simulink model "FaceDet_x4"  (Simulink 7.7)
settings: Solver=FixedStepDiscrete  StartTime=0  StopTime=10  RelTol=1e-3
libraries: simulink x257
(part 2 of 5)

== system FaceDet_x4/FaceDetection/FU/MemBank ==
  LineIdxsLatch : Inport
  LineIdxsExt : Inport  Port=2
  NodeWeightsCtrlRdAdr : Inport  Port=3
  NodeWeightsCtrlWrAdr : Inport  Port=4
  NodeWeightsCtrlEn : Inport  Port=5
  NodeWeightsExt : Inport  Port=6
  FeatureDataLatch : Inport  Port=7
  FeatureDataExt : Inport  Port=8
  WeakTreshLatch : Inport  Port=9
  WeakTreshExt : Inport  Port=10
  StrongTreshLatch : Inport  Port=11
  StrongTreshExt : Inport  Port=12
  FeatureDataMem : Subsystem
  LineIdxsMem : Subsystem
  NodeWeightsMem : Subsystem
  StrongTreshReg : simulink/Additional Math & Discrete/Additional Discrete/Unit Delay Enabled  SystemSampleTime=-1  vinit=0  tsamp=-1
  WeakTreshMem : Subsystem
  LineIdxs : Outport
  NodeWeights : Outport  Port=2
  FeatureData : Outport  Port=3
  StrongTresh : Outport  Port=4
  WeakTresh : Outport  Port=5
  wires:
  LineIdxsLatch/1 -> LineIdxsMem/1(LineIdxsLatch)
  LineIdxsExt/1 -> LineIdxsMem/2(LineIdxsExt)
  LineIdxsMem/1(LineIdxs) -> LineIdxs/1
  NodeWeightsCtrlRdAdr/1 -> NodeWeightsMem/1(NodeWeightsCtrlRdAdr)
  NodeWeightsExt/1 -> NodeWeightsMem/4(NodeWeightsExt)
  NodeWeightsMem/1(NodeWeights) -> NodeWeights/1
  FeatureDataMem/1(FeatureData) -> FeatureData/1
  FeatureDataLatch/1 -> FeatureDataMem/1(FeatureDataLatch)
  FeatureDataExt/1 -> FeatureDataMem/2(FeatureDataExt)
  WeakTreshMem/1(WeakTresh) -> WeakTresh/1
  WeakTreshLatch/1 -> WeakTreshMem/1(WeakTreshLatch)
  WeakTreshExt/1 -> WeakTreshMem/2(WeakTreshExt)
  StrongTreshReg/1 -> StrongTresh/1
  NodeWeightsCtrlEn/1 -> NodeWeightsMem/3(NodeWeightsCtrlEn)
  StrongTreshLatch/1 -> StrongTreshReg/2
  StrongTreshExt/1 -> StrongTreshReg/1
  NodeWeightsCtrlWrAdr/1 -> NodeWeightsMem/2(NodeWeightsCtrlWrAdr)

== system FaceDet_x4/FaceDetection/DU/SplittedDL1/DelLine0_SPRAM_512x5 ==
  addr : Inport
  din : Inport  Port=2
  we : Inport  Port=3  OutDataTypeStr=boolean
  AddressSpec : SignalSpecification  OutDataTypeStr=fixdt(0,depth_bits,0)  Dimensions=1
  And : Logic  AllPortsSameDT=off  OutDataTypeStr=boolean
  DataSpec : SignalSpecification  OutDataTypeStr=fixdt(0,width_bits,0)  Dimensions=1
  Switch1 : Switch  Criteria=u2 ~= 0
  convert : DataTypeConversion  OutDataTypeStr=uint16
  din_d : UnitDelay  SampleTime=-1
  dout_type : Constant  Value=dout_type
  is_new : simulink/Logic and Bit Operations/Compare To Constant  SystemSampleTime=-1  relop===  const=1  LogicOutDataTypeMode=boolean  ZeroCross=off
  ram : UnitDelay  SampleTime=-1
  ram_data : UnitDelay  SampleTime=-1
  select : Selector  IndexMode=Zero-based  InputPortWidth=2^depth_bits  IndexOptions=Index vector (port)  Indices=[1 3]  OutputSizes=1
  switch : Switch  Criteria=u2 ~= 0
  we_d : UnitDelay  SampleTime=-1
  wr_port : Assignment  IndexMode=Zero-based  IndexOptions=Index vector (port)  Indices=1  OutputSizes=[1 1]
  dout : Outport
  wires:
  wr_port/1 -> switch/1
  switch/1 -> ram/1
  ram/1 -> switch/3, wr_port/1, select/1
  din/1 -> DataSpec/1
  we/1 -> switch/2, we_d/1
  addr/1 -> AddressSpec/1
  select/1 -> ram_data/1
  convert/1 -> wr_port/3, select/2
  AddressSpec/1 -> convert/1
  Switch1/1 -> dout/1
  din_d/1 -> Switch1/1
  And/1 -> Switch1/2
  ram_data/1 -> Switch1/3
  dout_type/1 -> is_new/1
  is_new/1 -> And/2
  we_d/1 -> And/1
  DataSpec/1 -> wr_port/2, din_d/1

== system FaceDet_x4/FaceDetection/DU/SplittedDL1/DelLine1_SPRAM_512x5 ==
  addr : Inport
  din : Inport  Port=2
  we : Inport  Port=3  OutDataTypeStr=boolean
  AddressSpec : SignalSpecification  OutDataTypeStr=fixdt(0,depth_bits,0)  Dimensions=1
  And : Logic  AllPortsSameDT=off  OutDataTypeStr=boolean
  DataSpec : SignalSpecification  OutDataTypeStr=fixdt(0,width_bits,0)  Dimensions=1
  Switch1 : Switch  Criteria=u2 ~= 0
  convert : DataTypeConversion  OutDataTypeStr=uint16
  din_d : UnitDelay  SampleTime=-1
  dout_type : Constant  Value=dout_type
  is_new : simulink/Logic and Bit Operations/Compare To Constant  SystemSampleTime=-1  relop===  const=1  LogicOutDataTypeMode=boolean  ZeroCross=off
  ram : UnitDelay  SampleTime=-1
  ram_data : UnitDelay  SampleTime=-1
  select : Selector  IndexMode=Zero-based  InputPortWidth=2^depth_bits  IndexOptions=Index vector (port)  Indices=[1 3]  OutputSizes=1
  switch : Switch  Criteria=u2 ~= 0
  we_d : UnitDelay  SampleTime=-1
  wr_port : Assignment  IndexMode=Zero-based  IndexOptions=Index vector (port)  Indices=1  OutputSizes=[1 1]
  dout : Outport
  wires:
  DataSpec/1 -> din_d/1, wr_port/2
  we_d/1 -> And/1
  is_new/1 -> And/2
  dout_type/1 -> is_new/1
  ram_data/1 -> Switch1/3
  And/1 -> Switch1/2
  din_d/1 -> Switch1/1
  Switch1/1 -> dout/1
  AddressSpec/1 -> convert/1
  convert/1 -> select/2, wr_port/3
  select/1 -> ram_data/1
  addr/1 -> AddressSpec/1
  we/1 -> we_d/1, switch/2
  din/1 -> DataSpec/1
  ram/1 -> select/1, wr_port/1, switch/3
  switch/1 -> ram/1
  wr_port/1 -> switch/1

== system FaceDet_x4/FaceDetection/DU/SplittedDL1/DelLine2_SPRAM_512x5 ==
  addr : Inport
  din : Inport  Port=2
  we : Inport  Port=3  OutDataTypeStr=boolean
  AddressSpec : SignalSpecification  OutDataTypeStr=fixdt(0,depth_bits,0)  Dimensions=1
  And : Logic  AllPortsSameDT=off  OutDataTypeStr=boolean
  DataSpec : SignalSpecification  OutDataTypeStr=fixdt(0,width_bits,0)  Dimensions=1
  Switch1 : Switch  Criteria=u2 ~= 0
  convert : DataTypeConversion  OutDataTypeStr=uint16
  din_d : UnitDelay  SampleTime=-1
  dout_type : Constant  Value=dout_type
  is_new : simulink/Logic and Bit Operations/Compare To Constant  SystemSampleTime=-1  relop===  const=1  LogicOutDataTypeMode=boolean  ZeroCross=off
  ram : UnitDelay  SampleTime=-1
  ram_data : UnitDelay  SampleTime=-1
  select : Selector  IndexMode=Zero-based  InputPortWidth=2^depth_bits  IndexOptions=Index vector (port)  Indices=[1 3]  OutputSizes=1
  switch : Switch  Criteria=u2 ~= 0
  we_d : UnitDelay  SampleTime=-1
  wr_port : Assignment  IndexMode=Zero-based  IndexOptions=Index vector (port)  Indices=1  OutputSizes=[1 1]
  dout : Outport
  wires:
  wr_port/1 -> switch/1
  switch/1 -> ram/1
  ram/1 -> switch/3, wr_port/1, select/1
  din/1 -> DataSpec/1
  we/1 -> switch/2, we_d/1
  addr/1 -> AddressSpec/1
  select/1 -> ram_data/1
  convert/1 -> wr_port/3, select/2
  AddressSpec/1 -> convert/1
  Switch1/1 -> dout/1
  din_d/1 -> Switch1/1
  And/1 -> Switch1/2
  ram_data/1 -> Switch1/3
  dout_type/1 -> is_new/1
  is_new/1 -> And/2
  we_d/1 -> And/1
  DataSpec/1 -> wr_port/2, din_d/1

== system FaceDet_x4/FaceDetection/DU/SplittedDL1/DelLine3_SPRAM_512x5 ==
  addr : Inport
  din : Inport  Port=2
  we : Inport  Port=3  OutDataTypeStr=boolean
  AddressSpec : SignalSpecification  OutDataTypeStr=fixdt(0,depth_bits,0)  Dimensions=1
  And : Logic  AllPortsSameDT=off  OutDataTypeStr=boolean
  DataSpec : SignalSpecification  OutDataTypeStr=fixdt(0,width_bits,0)  Dimensions=1
  Switch1 : Switch  Criteria=u2 ~= 0
  convert : DataTypeConversion  OutDataTypeStr=uint16
  din_d : UnitDelay  SampleTime=-1
  dout_type : Constant  Value=dout_type
  is_new : simulink/Logic and Bit Operations/Compare To Constant  SystemSampleTime=-1  relop===  const=1  LogicOutDataTypeMode=boolean  ZeroCross=off
  ram : UnitDelay  SampleTime=-1
  ram_data : UnitDelay  SampleTime=-1
  select : Selector  IndexMode=Zero-based  InputPortWidth=2^depth_bits  IndexOptions=Index vector (port)  Indices=[1 3]  OutputSizes=1
  switch : Switch  Criteria=u2 ~= 0
  we_d : UnitDelay  SampleTime=-1
  wr_port : Assignment  IndexMode=Zero-based  IndexOptions=Index vector (port)  Indices=1  OutputSizes=[1 1]
  dout : Outport
  wires:
  DataSpec/1 -> din_d/1, wr_port/2
  we_d/1 -> And/1
  is_new/1 -> And/2
  dout_type/1 -> is_new/1
  ram_data/1 -> Switch1/3
  And/1 -> Switch1/2
  din_d/1 -> Switch1/1
  Switch1/1 -> dout/1
  AddressSpec/1 -> convert/1
  convert/1 -> select/2, wr_port/3
  select/1 -> ram_data/1
  addr/1 -> AddressSpec/1
  we/1 -> we_d/1, switch/2
  din/1 -> DataSpec/1
  ram/1 -> select/1, wr_port/1, switch/3
  switch/1 -> ram/1
  wr_port/1 -> switch/1

== system FaceDet_x4/FaceDetection/DU/SplittedDL1/DelLine4_SPRAM_512x5 ==
  addr : Inport
  din : Inport  Port=2
  we : Inport  Port=3  OutDataTypeStr=boolean
  AddressSpec : SignalSpecification  OutDataTypeStr=fixdt(0,depth_bits,0)  Dimensions=1
  And : Logic  AllPortsSameDT=off  OutDataTypeStr=boolean
  DataSpec : SignalSpecification  OutDataTypeStr=fixdt(0,width_bits,0)  Dimensions=1
  Switch1 : Switch  Criteria=u2 ~= 0
  convert : DataTypeConversion  OutDataTypeStr=uint16
  din_d : UnitDelay  SampleTime=-1
  dout_type : Constant  Value=dout_type
  is_new : simulink/Logic and Bit Operations/Compare To Constant  SystemSampleTime=-1  relop===  const=1  LogicOutDataTypeMode=boolean  ZeroCross=off
  ram : UnitDelay  SampleTime=-1
  ram_data : UnitDelay  SampleTime=-1
  select : Selector  IndexMode=Zero-based  InputPortWidth=2^depth_bits  IndexOptions=Index vector (port)  Indices=[1 3]  OutputSizes=1
  switch : Switch  Criteria=u2 ~= 0
  we_d : UnitDelay  SampleTime=-1
  wr_port : Assignment  IndexMode=Zero-based  IndexOptions=Index vector (port)  Indices=1  OutputSizes=[1 1]
  dout : Outport
  wires:
  wr_port/1 -> switch/1
  switch/1 -> ram/1
  ram/1 -> switch/3, wr_port/1, select/1
  din/1 -> DataSpec/1
  we/1 -> switch/2, we_d/1
  addr/1 -> AddressSpec/1
  select/1 -> ram_data/1
  convert/1 -> wr_port/3, select/2
  AddressSpec/1 -> convert/1
  Switch1/1 -> dout/1
  din_d/1 -> Switch1/1
  And/1 -> Switch1/2
  ram_data/1 -> Switch1/3
  dout_type/1 -> is_new/1
  is_new/1 -> And/2
  we_d/1 -> And/1
  DataSpec/1 -> wr_port/2, din_d/1

== system FaceDet_x4/FaceDetection/DU/SplittedDL1/DelLine5_SPRAM_512x5 ==
  addr : Inport
  din : Inport  Port=2
  we : Inport  Port=3  OutDataTypeStr=boolean
  AddressSpec : SignalSpecification  OutDataTypeStr=fixdt(0,depth_bits,0)  Dimensions=1
  And : Logic  AllPortsSameDT=off  OutDataTypeStr=boolean
  DataSpec : SignalSpecification  OutDataTypeStr=fixdt(0,width_bits,0)  Dimensions=1
  Switch1 : Switch  Criteria=u2 ~= 0
  convert : DataTypeConversion  OutDataTypeStr=uint16
  din_d : UnitDelay  SampleTime=-1
  dout_type : Constant  Value=dout_type
  is_new : simulink/Logic and Bit Operations/Compare To Constant  SystemSampleTime=-1  relop===  const=1  LogicOutDataTypeMode=boolean  ZeroCross=off
  ram : UnitDelay  SampleTime=-1
  ram_data : UnitDelay  SampleTime=-1
  select : Selector  IndexMode=Zero-based  InputPortWidth=2^depth_bits  IndexOptions=Index vector (port)  Indices=[1 3]  OutputSizes=1
  switch : Switch  Criteria=u2 ~= 0
  we_d : UnitDelay  SampleTime=-1
  wr_port : Assignment  IndexMode=Zero-based  IndexOptions=Index vector (port)  Indices=1  OutputSizes=[1 1]
  dout : Outport
  wires:
  DataSpec/1 -> din_d/1, wr_port/2
  we_d/1 -> And/1
  is_new/1 -> And/2
  dout_type/1 -> is_new/1
  ram_data/1 -> Switch1/3
  And/1 -> Switch1/2
  din_d/1 -> Switch1/1
  Switch1/1 -> dout/1
  AddressSpec/1 -> convert/1
  convert/1 -> select/2, wr_port/3
  select/1 -> ram_data/1
  addr/1 -> AddressSpec/1
  we/1 -> we_d/1, switch/2
  din/1 -> DataSpec/1
  ram/1 -> select/1, wr_port/1, switch/3
  switch/1 -> ram/1
  wr_port/1 -> switch/1

== system FaceDet_x4/FaceDetection/DU/SplittedDL1/DelLine6_SPRAM_512x5 ==
  addr : Inport
  din : Inport  Port=2
  we : Inport  Port=3  OutDataTypeStr=boolean
  AddressSpec : SignalSpecification  OutDataTypeStr=fixdt(0,depth_bits,0)  Dimensions=1
  And : Logic  AllPortsSameDT=off  OutDataTypeStr=boolean
  DataSpec : SignalSpecification  OutDataTypeStr=fixdt(0,width_bits,0)  Dimensions=1
  Switch1 : Switch  Criteria=u2 ~= 0
  convert : DataTypeConversion  OutDataTypeStr=uint16
  din_d : UnitDelay  SampleTime=-1
  dout_type : Constant  Value=dout_type
  is_new : simulink/Logic and Bit Operations/Compare To Constant  SystemSampleTime=-1  relop===  const=1  LogicOutDataTypeMode=boolean  ZeroCross=off
  ram : UnitDelay  SampleTime=-1
  ram_data : UnitDelay  SampleTime=-1
  select : Selector  IndexMode=Zero-based  InputPortWidth=2^depth_bits  IndexOptions=Index vector (port)  Indices=[1 3]  OutputSizes=1
  switch : Switch  Criteria=u2 ~= 0
  we_d : UnitDelay  SampleTime=-1
  wr_port : Assignment  IndexMode=Zero-based  IndexOptions=Index vector (port)  Indices=1  OutputSizes=[1 1]
  dout : Outport
  wires:
  DataSpec/1 -> din_d/1, wr_port/2
  we_d/1 -> And/1
  is_new/1 -> And/2
  dout_type/1 -> is_new/1
  ram_data/1 -> Switch1/3
  And/1 -> Switch1/2
  din_d/1 -> Switch1/1
  Switch1/1 -> dout/1
  AddressSpec/1 -> convert/1
  convert/1 -> select/2, wr_port/3
  select/1 -> ram_data/1
  addr/1 -> AddressSpec/1
  we/1 -> we_d/1, switch/2
  din/1 -> DataSpec/1
  ram/1 -> select/1, wr_port/1, switch/3
  switch/1 -> ram/1
  wr_port/1 -> switch/1

== system FaceDet_x4/FaceDetection/DU/SplittedDL1/DelLine7_SPRAM_512x5 ==
  addr : Inport
  din : Inport  Port=2
  we : Inport  Port=3  OutDataTypeStr=boolean
  AddressSpec : SignalSpecification  OutDataTypeStr=fixdt(0,depth_bits,0)  Dimensions=1
  And : Logic  AllPortsSameDT=off  OutDataTypeStr=boolean
  DataSpec : SignalSpecification  OutDataTypeStr=fixdt(0,width_bits,0)  Dimensions=1
  Switch1 : Switch  Criteria=u2 ~= 0
  convert : DataTypeConversion  OutDataTypeStr=uint16
  din_d : UnitDelay  SampleTime=-1
  dout_type : Constant  Value=dout_type
  is_new : simulink/Logic and Bit Operations/Compare To Constant  SystemSampleTime=-1  relop===  const=1  LogicOutDataTypeMode=boolean  ZeroCross=off
  ram : UnitDelay  SampleTime=-1
  ram_data : UnitDelay  SampleTime=-1
  select : Selector  IndexMode=Zero-based  InputPortWidth=2^depth_bits  IndexOptions=Index vector (port)  Indices=[1 3]  OutputSizes=1
  switch : Switch  Criteria=u2 ~= 0
  we_d : UnitDelay  SampleTime=-1
  wr_port : Assignment  IndexMode=Zero-based  IndexOptions=Index vector (port)  Indices=1  OutputSizes=[1 1]
  dout : Outport
  wires:
  wr_port/1 -> switch/1
  switch/1 -> ram/1
  ram/1 -> switch/3, wr_port/1, select/1
  din/1 -> DataSpec/1
  we/1 -> switch/2, we_d/1
  addr/1 -> AddressSpec/1
  select/1 -> ram_data/1
  convert/1 -> wr_port/3, select/2
  AddressSpec/1 -> convert/1
  Switch1/1 -> dout/1
  din_d/1 -> Switch1/1
  And/1 -> Switch1/2
  ram_data/1 -> Switch1/3
  dout_type/1 -> is_new/1
  is_new/1 -> And/2
  we_d/1 -> And/1
  DataSpec/1 -> wr_port/2, din_d/1

== system FaceDet_x4/FaceDetection/DU/SplittedDL2/DelLine0_SPRAM_512x5 ==
  addr : Inport
  din : Inport  Port=2
  we : Inport  Port=3  OutDataTypeStr=boolean
  AddressSpec : SignalSpecification  OutDataTypeStr=fixdt(0,depth_bits,0)  Dimensions=1
  And : Logic  AllPortsSameDT=off  OutDataTypeStr=boolean
  DataSpec : SignalSpecification  OutDataTypeStr=fixdt(0,width_bits,0)  Dimensions=1
  Switch1 : Switch  Criteria=u2 ~= 0
  convert : DataTypeConversion  OutDataTypeStr=uint16
  din_d : UnitDelay  SampleTime=-1
  dout_type : Constant  Value=dout_type
  is_new : simulink/Logic and Bit Operations/Compare To Constant  SystemSampleTime=-1  relop===  const=1  LogicOutDataTypeMode=boolean  ZeroCross=off
  ram : UnitDelay  SampleTime=-1
  ram_data : UnitDelay  SampleTime=-1
  select : Selector  IndexMode=Zero-based  InputPortWidth=2^depth_bits  IndexOptions=Index vector (port)  Indices=[1 3]  OutputSizes=1
  switch : Switch  Criteria=u2 ~= 0
  we_d : UnitDelay  SampleTime=-1
  wr_port : Assignment  IndexMode=Zero-based  IndexOptions=Index vector (port)  Indices=1  OutputSizes=[1 1]
  dout : Outport
  wires:
  DataSpec/1 -> din_d/1, wr_port/2
  we_d/1 -> And/1
  is_new/1 -> And/2
  dout_type/1 -> is_new/1
  ram_data/1 -> Switch1/3
  And/1 -> Switch1/2
  din_d/1 -> Switch1/1
  Switch1/1 -> dout/1
  AddressSpec/1 -> convert/1
  convert/1 -> select/2, wr_port/3
  select/1 -> ram_data/1
  addr/1 -> AddressSpec/1
  we/1 -> we_d/1, switch/2
  din/1 -> DataSpec/1
  ram/1 -> select/1, wr_port/1, switch/3
  switch/1 -> ram/1
  wr_port/1 -> switch/1

== system FaceDet_x4/FaceDetection/DU/SplittedDL2/DelLine1_SPRAM_512x5 ==
  addr : Inport
  din : Inport  Port=2
  we : Inport  Port=3  OutDataTypeStr=boolean
  AddressSpec : SignalSpecification  OutDataTypeStr=fixdt(0,depth_bits,0)  Dimensions=1
  And : Logic  AllPortsSameDT=off  OutDataTypeStr=boolean
  DataSpec : SignalSpecification  OutDataTypeStr=fixdt(0,width_bits,0)  Dimensions=1
  Switch1 : Switch  Criteria=u2 ~= 0
  convert : DataTypeConversion  OutDataTypeStr=uint16
  din_d : UnitDelay  SampleTime=-1
  dout_type : Constant  Value=dout_type
  is_new : simulink/Logic and Bit Operations/Compare To Constant  SystemSampleTime=-1  relop===  const=1  LogicOutDataTypeMode=boolean  ZeroCross=off
  ram : UnitDelay  SampleTime=-1
  ram_data : UnitDelay  SampleTime=-1
  select : Selector  IndexMode=Zero-based  InputPortWidth=2^depth_bits  IndexOptions=Index vector (port)  Indices=[1 3]  OutputSizes=1
  switch : Switch  Criteria=u2 ~= 0
  we_d : UnitDelay  SampleTime=-1
  wr_port : Assignment  IndexMode=Zero-based  IndexOptions=Index vector (port)  Indices=1  OutputSizes=[1 1]
  dout : Outport
  wires:
  wr_port/1 -> switch/1
  switch/1 -> ram/1
  ram/1 -> switch/3, wr_port/1, select/1
  din/1 -> DataSpec/1
  we/1 -> switch/2, we_d/1
  addr/1 -> AddressSpec/1
  select/1 -> ram_data/1
  convert/1 -> wr_port/3, select/2
  AddressSpec/1 -> convert/1
  Switch1/1 -> dout/1
  din_d/1 -> Switch1/1
  And/1 -> Switch1/2
  ram_data/1 -> Switch1/3
  dout_type/1 -> is_new/1
  is_new/1 -> And/2
  we_d/1 -> And/1
  DataSpec/1 -> wr_port/2, din_d/1

== system FaceDet_x4/FaceDetection/DU/SplittedDL2/DelLine2_SPRAM_512x5 ==
  addr : Inport
  din : Inport  Port=2
  we : Inport  Port=3  OutDataTypeStr=boolean
  AddressSpec : SignalSpecification  OutDataTypeStr=fixdt(0,depth_bits,0)  Dimensions=1
  And : Logic  AllPortsSameDT=off  OutDataTypeStr=boolean
  DataSpec : SignalSpecification  OutDataTypeStr=fixdt(0,width_bits,0)  Dimensions=1
  Switch1 : Switch  Criteria=u2 ~= 0
  convert : DataTypeConversion  OutDataTypeStr=uint16
  din_d : UnitDelay  SampleTime=-1
  dout_type : Constant  Value=dout_type
  is_new : simulink/Logic and Bit Operations/Compare To Constant  SystemSampleTime=-1  relop===  const=1  LogicOutDataTypeMode=boolean  ZeroCross=off
  ram : UnitDelay  SampleTime=-1
  ram_data : UnitDelay  SampleTime=-1
  select : Selector  IndexMode=Zero-based  InputPortWidth=2^depth_bits  IndexOptions=Index vector (port)  Indices=[1 3]  OutputSizes=1
  switch : Switch  Criteria=u2 ~= 0
  we_d : UnitDelay  SampleTime=-1
  wr_port : Assignment  IndexMode=Zero-based  IndexOptions=Index vector (port)  Indices=1  OutputSizes=[1 1]
  dout : Outport
  wires:
  DataSpec/1 -> din_d/1, wr_port/2
  we_d/1 -> And/1
  is_new/1 -> And/2
  dout_type/1 -> is_new/1
  ram_data/1 -> Switch1/3
  And/1 -> Switch1/2
  din_d/1 -> Switch1/1
  Switch1/1 -> dout/1
  AddressSpec/1 -> convert/1
  convert/1 -> select/2, wr_port/3
  select/1 -> ram_data/1
  addr/1 -> AddressSpec/1
  we/1 -> we_d/1, switch/2
  din/1 -> DataSpec/1
  ram/1 -> select/1, wr_port/1, switch/3
  switch/1 -> ram/1
  wr_port/1 -> switch/1

== system FaceDet_x4/FaceDetection/DU/SplittedDL2/DelLine3_SPRAM_512x5 ==
  addr : Inport
  din : Inport  Port=2
  we : Inport  Port=3  OutDataTypeStr=boolean
  AddressSpec : SignalSpecification  OutDataTypeStr=fixdt(0,depth_bits,0)  Dimensions=1
  And : Logic  AllPortsSameDT=off  OutDataTypeStr=boolean
  DataSpec : SignalSpecification  OutDataTypeStr=fixdt(0,width_bits,0)  Dimensions=1
  Switch1 : Switch  Criteria=u2 ~= 0
  convert : DataTypeConversion  OutDataTypeStr=uint16
  din_d : UnitDelay  SampleTime=-1
  dout_type : Constant  Value=dout_type
  is_new : simulink/Logic and Bit Operations/Compare To Constant  SystemSampleTime=-1  relop===  const=1  LogicOutDataTypeMode=boolean  ZeroCross=off
  ram : UnitDelay  SampleTime=-1
  ram_data : UnitDelay  SampleTime=-1
  select : Selector  IndexMode=Zero-based  InputPortWidth=2^depth_bits  IndexOptions=Index vector (port)  Indices=[1 3]  OutputSizes=1
  switch : Switch  Criteria=u2 ~= 0
  we_d : UnitDelay  SampleTime=-1
  wr_port : Assignment  IndexMode=Zero-based  IndexOptions=Index vector (port)  Indices=1  OutputSizes=[1 1]
  dout : Outport
  wires:
  wr_port/1 -> switch/1
  switch/1 -> ram/1
  ram/1 -> switch/3, wr_port/1, select/1
  din/1 -> DataSpec/1
  we/1 -> switch/2, we_d/1
  addr/1 -> AddressSpec/1
  select/1 -> ram_data/1
  convert/1 -> wr_port/3, select/2
  AddressSpec/1 -> convert/1
  Switch1/1 -> dout/1
  din_d/1 -> Switch1/1
  And/1 -> Switch1/2
  ram_data/1 -> Switch1/3
  dout_type/1 -> is_new/1
  is_new/1 -> And/2
  we_d/1 -> And/1
  DataSpec/1 -> wr_port/2, din_d/1

== system FaceDet_x4/FaceDetection/DU/SplittedDL2/DelLine4_SPRAM_512x5 ==
  addr : Inport
  din : Inport  Port=2
  we : Inport  Port=3  OutDataTypeStr=boolean
  AddressSpec : SignalSpecification  OutDataTypeStr=fixdt(0,depth_bits,0)  Dimensions=1
  And : Logic  AllPortsSameDT=off  OutDataTypeStr=boolean
  DataSpec : SignalSpecification  OutDataTypeStr=fixdt(0,width_bits,0)  Dimensions=1
  Switch1 : Switch  Criteria=u2 ~= 0
  convert : DataTypeConversion  OutDataTypeStr=uint16
  din_d : UnitDelay  SampleTime=-1
  dout_type : Constant  Value=dout_type
  is_new : simulink/Logic and Bit Operations/Compare To Constant  SystemSampleTime=-1  relop===  const=1  LogicOutDataTypeMode=boolean  ZeroCross=off
  ram : UnitDelay  SampleTime=-1
  ram_data : UnitDelay  SampleTime=-1
  select : Selector  IndexMode=Zero-based  InputPortWidth=2^depth_bits  IndexOptions=Index vector (port)  Indices=[1 3]  OutputSizes=1
  switch : Switch  Criteria=u2 ~= 0
  we_d : UnitDelay  SampleTime=-1
  wr_port : Assignment  IndexMode=Zero-based  IndexOptions=Index vector (port)  Indices=1  OutputSizes=[1 1]
  dout : Outport
  wires:
  DataSpec/1 -> din_d/1, wr_port/2
  we_d/1 -> And/1
  is_new/1 -> And/2
  dout_type/1 -> is_new/1
  ram_data/1 -> Switch1/3
  And/1 -> Switch1/2
  din_d/1 -> Switch1/1
  Switch1/1 -> dout/1
  AddressSpec/1 -> convert/1
  convert/1 -> select/2, wr_port/3
  select/1 -> ram_data/1
  addr/1 -> AddressSpec/1
  we/1 -> we_d/1, switch/2
  din/1 -> DataSpec/1
  ram/1 -> select/1, wr_port/1, switch/3
  switch/1 -> ram/1
  wr_port/1 -> switch/1

== system FaceDet_x4/FaceDetection/DU/SplittedDL2/DelLine5_SPRAM_512x5 ==
  addr : Inport
  din : Inport  Port=2
  we : Inport  Port=3  OutDataTypeStr=boolean
  AddressSpec : SignalSpecification  OutDataTypeStr=fixdt(0,depth_bits,0)  Dimensions=1
  And : Logic  AllPortsSameDT=off  OutDataTypeStr=boolean
  DataSpec : SignalSpecification  OutDataTypeStr=fixdt(0,width_bits,0)  Dimensions=1
  Switch1 : Switch  Criteria=u2 ~= 0
  convert : DataTypeConversion  OutDataTypeStr=uint16
  din_d : UnitDelay  SampleTime=-1
  dout_type : Constant  Value=dout_type
  is_new : simulink/Logic and Bit Operations/Compare To Constant  SystemSampleTime=-1  relop===  const=1  LogicOutDataTypeMode=boolean  ZeroCross=off
  ram : UnitDelay  SampleTime=-1
  ram_data : UnitDelay  SampleTime=-1
  select : Selector  IndexMode=Zero-based  InputPortWidth=2^depth_bits  IndexOptions=Index vector (port)  Indices=[1 3]  OutputSizes=1
  switch : Switch  Criteria=u2 ~= 0
  we_d : UnitDelay  SampleTime=-1
  wr_port : Assignment  IndexMode=Zero-based  IndexOptions=Index vector (port)  Indices=1  OutputSizes=[1 1]
  dout : Outport
  wires:
  wr_port/1 -> switch/1
  switch/1 -> ram/1
  ram/1 -> switch/3, wr_port/1, select/1
  din/1 -> DataSpec/1
  we/1 -> switch/2, we_d/1
  addr/1 -> AddressSpec/1
  select/1 -> ram_data/1
  convert/1 -> wr_port/3, select/2
  AddressSpec/1 -> convert/1
  Switch1/1 -> dout/1
  din_d/1 -> Switch1/1
  And/1 -> Switch1/2
  ram_data/1 -> Switch1/3
  dout_type/1 -> is_new/1
  is_new/1 -> And/2
  we_d/1 -> And/1
  DataSpec/1 -> wr_port/2, din_d/1

== system FaceDet_x4/FaceDetection/DU/SplittedDL2/DelLine6_SPRAM_512x5 ==
  addr : Inport
  din : Inport  Port=2
  we : Inport  Port=3  OutDataTypeStr=boolean
  AddressSpec : SignalSpecification  OutDataTypeStr=fixdt(0,depth_bits,0)  Dimensions=1
  And : Logic  AllPortsSameDT=off  OutDataTypeStr=boolean
  DataSpec : SignalSpecification  OutDataTypeStr=fixdt(0,width_bits,0)  Dimensions=1
  Switch1 : Switch  Criteria=u2 ~= 0
  convert : DataTypeConversion  OutDataTypeStr=uint16
  din_d : UnitDelay  SampleTime=-1
  dout_type : Constant  Value=dout_type
  is_new : simulink/Logic and Bit Operations/Compare To Constant  SystemSampleTime=-1  relop===  const=1  LogicOutDataTypeMode=boolean  ZeroCross=off
  ram : UnitDelay  SampleTime=-1
  ram_data : UnitDelay  SampleTime=-1
  select : Selector  IndexMode=Zero-based  InputPortWidth=2^depth_bits  IndexOptions=Index vector (port)  Indices=[1 3]  OutputSizes=1
  switch : Switch  Criteria=u2 ~= 0
  we_d : UnitDelay  SampleTime=-1
  wr_port : Assignment  IndexMode=Zero-based  IndexOptions=Index vector (port)  Indices=1  OutputSizes=[1 1]
  dout : Outport
  wires:
  wr_port/1 -> switch/1
  switch/1 -> ram/1
  ram/1 -> switch/3, wr_port/1, select/1
  din/1 -> DataSpec/1
  we/1 -> switch/2, we_d/1
  addr/1 -> AddressSpec/1
  select/1 -> ram_data/1
  convert/1 -> wr_port/3, select/2
  AddressSpec/1 -> convert/1
  Switch1/1 -> dout/1
  din_d/1 -> Switch1/1
  And/1 -> Switch1/2
  ram_data/1 -> Switch1/3
  dout_type/1 -> is_new/1
  is_new/1 -> And/2
  we_d/1 -> And/1
  DataSpec/1 -> wr_port/2, din_d/1

== system FaceDet_x4/FaceDetection/DU/SplittedDL2/DelLine7_SPRAM_512x5 ==
  addr : Inport
  din : Inport  Port=2
  we : Inport  Port=3  OutDataTypeStr=boolean
  AddressSpec : SignalSpecification  OutDataTypeStr=fixdt(0,depth_bits,0)  Dimensions=1
  And : Logic  AllPortsSameDT=off  OutDataTypeStr=boolean
  DataSpec : SignalSpecification  OutDataTypeStr=fixdt(0,width_bits,0)  Dimensions=1
  Switch1 : Switch  Criteria=u2 ~= 0
  convert : DataTypeConversion  OutDataTypeStr=uint16
  din_d : UnitDelay  SampleTime=-1
  dout_type : Constant  Value=dout_type
  is_new : simulink/Logic and Bit Operations/Compare To Constant  SystemSampleTime=-1  relop===  const=1  LogicOutDataTypeMode=boolean  ZeroCross=off
  ram : UnitDelay  SampleTime=-1
  ram_data : UnitDelay  SampleTime=-1
  select : Selector  IndexMode=Zero-based  InputPortWidth=2^depth_bits  IndexOptions=Index vector (port)  Indices=[1 3]  OutputSizes=1
  switch : Switch  Criteria=u2 ~= 0
  we_d : UnitDelay  SampleTime=-1
  wr_port : Assignment  IndexMode=Zero-based  IndexOptions=Index vector (port)  Indices=1  OutputSizes=[1 1]
  dout : Outport
  wires:
  DataSpec/1 -> din_d/1, wr_port/2
  we_d/1 -> And/1
  is_new/1 -> And/2
  dout_type/1 -> is_new/1
  ram_data/1 -> Switch1/3
  And/1 -> Switch1/2
  din_d/1 -> Switch1/1
  Switch1/1 -> dout/1
  AddressSpec/1 -> convert/1
  convert/1 -> select/2, wr_port/3
  select/1 -> ram_data/1
  addr/1 -> AddressSpec/1
  we/1 -> we_d/1, switch/2
  din/1 -> DataSpec/1
  ram/1 -> select/1, wr_port/1, switch/3
  switch/1 -> ram/1
  wr_port/1 -> switch/1

== system FaceDet_x4/FaceDetection/DU/SplittedDL3/DelLine0_SPRAM_512x5 ==
  addr : Inport
  din : Inport  Port=2
  we : Inport  Port=3  OutDataTypeStr=boolean
  AddressSpec : SignalSpecification  OutDataTypeStr=fixdt(0,depth_bits,0)  Dimensions=1
  And : Logic  AllPortsSameDT=off  OutDataTypeStr=boolean
  DataSpec : SignalSpecification  OutDataTypeStr=fixdt(0,width_bits,0)  Dimensions=1
  Switch1 : Switch  Criteria=u2 ~= 0
  convert : DataTypeConversion  OutDataTypeStr=uint16
  din_d : UnitDelay  SampleTime=-1
  dout_type : Constant  Value=dout_type
  is_new : simulink/Logic and Bit Operations/Compare To Constant  SystemSampleTime=-1  relop===  const=1  LogicOutDataTypeMode=boolean  ZeroCross=off
  ram : UnitDelay  SampleTime=-1
  ram_data : UnitDelay  SampleTime=-1
  select : Selector  IndexMode=Zero-based  InputPortWidth=2^depth_bits  IndexOptions=Index vector (port)  Indices=[1 3]  OutputSizes=1
  switch : Switch  Criteria=u2 ~= 0
  we_d : UnitDelay  SampleTime=-1
  wr_port : Assignment  IndexMode=Zero-based  IndexOptions=Index vector (port)  Indices=1  OutputSizes=[1 1]
  dout : Outport
  wires:
  wr_port/1 -> switch/1
  switch/1 -> ram/1
  ram/1 -> switch/3, wr_port/1, select/1
  din/1 -> DataSpec/1
  we/1 -> switch/2, we_d/1
  addr/1 -> AddressSpec/1
  select/1 -> ram_data/1
  convert/1 -> wr_port/3, select/2
  AddressSpec/1 -> convert/1
  Switch1/1 -> dout/1
  din_d/1 -> Switch1/1
  And/1 -> Switch1/2
  ram_data/1 -> Switch1/3
  dout_type/1 -> is_new/1
  is_new/1 -> And/2
  we_d/1 -> And/1
  DataSpec/1 -> wr_port/2, din_d/1

== system FaceDet_x4/FaceDetection/DU/SplittedDL3/DelLine1_SPRAM_512x5 ==
  addr : Inport
  din : Inport  Port=2
  we : Inport  Port=3  OutDataTypeStr=boolean
  AddressSpec : SignalSpecification  OutDataTypeStr=fixdt(0,depth_bits,0)  Dimensions=1
  And : Logic  AllPortsSameDT=off  OutDataTypeStr=boolean
  DataSpec : SignalSpecification  OutDataTypeStr=fixdt(0,width_bits,0)  Dimensions=1
  Switch1 : Switch  Criteria=u2 ~= 0
  convert : DataTypeConversion  OutDataTypeStr=uint16
  din_d : UnitDelay  SampleTime=-1
  dout_type : Constant  Value=dout_type
  is_new : simulink/Logic and Bit Operations/Compare To Constant  SystemSampleTime=-1  relop===  const=1  LogicOutDataTypeMode=boolean  ZeroCross=off
  ram : UnitDelay  SampleTime=-1
  ram_data : UnitDelay  SampleTime=-1
  select : Selector  IndexMode=Zero-based  InputPortWidth=2^depth_bits  IndexOptions=Index vector (port)  Indices=[1 3]  OutputSizes=1
  switch : Switch  Criteria=u2 ~= 0
  we_d : UnitDelay  SampleTime=-1
  wr_port : Assignment  IndexMode=Zero-based  IndexOptions=Index vector (port)  Indices=1  OutputSizes=[1 1]
  dout : Outport
  wires:
  DataSpec/1 -> din_d/1, wr_port/2
  we_d/1 -> And/1
  is_new/1 -> And/2
  dout_type/1 -> is_new/1
  ram_data/1 -> Switch1/3
  And/1 -> Switch1/2
  din_d/1 -> Switch1/1
  Switch1/1 -> dout/1
  AddressSpec/1 -> convert/1
  convert/1 -> select/2, wr_port/3
  select/1 -> ram_data/1
  addr/1 -> AddressSpec/1
  we/1 -> we_d/1, switch/2
  din/1 -> DataSpec/1
  ram/1 -> select/1, wr_port/1, switch/3
  switch/1 -> ram/1
  wr_port/1 -> switch/1

== system FaceDet_x4/FaceDetection/DU/SplittedDL3/DelLine2_SPRAM_512x5 ==
  addr : Inport
  din : Inport  Port=2
  we : Inport  Port=3  OutDataTypeStr=boolean
  AddressSpec : SignalSpecification  OutDataTypeStr=fixdt(0,depth_bits,0)  Dimensions=1
  And : Logic  AllPortsSameDT=off  OutDataTypeStr=boolean
  DataSpec : SignalSpecification  OutDataTypeStr=fixdt(0,width_bits,0)  Dimensions=1
  Switch1 : Switch  Criteria=u2 ~= 0
  convert : DataTypeConversion  OutDataTypeStr=uint16
  din_d : UnitDelay  SampleTime=-1
  dout_type : Constant  Value=dout_type
  is_new : simulink/Logic and Bit Operations/Compare To Constant  SystemSampleTime=-1  relop===  const=1  LogicOutDataTypeMode=boolean  ZeroCross=off
  ram : UnitDelay  SampleTime=-1
  ram_data : UnitDelay  SampleTime=-1
  select : Selector  IndexMode=Zero-based  InputPortWidth=2^depth_bits  IndexOptions=Index vector (port)  Indices=[1 3]  OutputSizes=1
  switch : Switch  Criteria=u2 ~= 0
  we_d : UnitDelay  SampleTime=-1
  wr_port : Assignment  IndexMode=Zero-based  IndexOptions=Index vector (port)  Indices=1  OutputSizes=[1 1]
  dout : Outport
  wires:
  wr_port/1 -> switch/1
  switch/1 -> ram/1
  ram/1 -> switch/3, wr_port/1, select/1
  din/1 -> DataSpec/1
  we/1 -> switch/2, we_d/1
  addr/1 -> AddressSpec/1
  select/1 -> ram_data/1
  convert/1 -> wr_port/3, select/2
  AddressSpec/1 -> convert/1
  Switch1/1 -> dout/1
  din_d/1 -> Switch1/1
  And/1 -> Switch1/2
  ram_data/1 -> Switch1/3
  dout_type/1 -> is_new/1
  is_new/1 -> And/2
  we_d/1 -> And/1
  DataSpec/1 -> wr_port/2, din_d/1

== system FaceDet_x4/FaceDetection/DU/SplittedDL3/DelLine3_SPRAM_512x5 ==
  addr : Inport
  din : Inport  Port=2
  we : Inport  Port=3  OutDataTypeStr=boolean
  AddressSpec : SignalSpecification  OutDataTypeStr=fixdt(0,depth_bits,0)  Dimensions=1
  And : Logic  AllPortsSameDT=off  OutDataTypeStr=boolean
  DataSpec : SignalSpecification  OutDataTypeStr=fixdt(0,width_bits,0)  Dimensions=1
  Switch1 : Switch  Criteria=u2 ~= 0
  convert : DataTypeConversion  OutDataTypeStr=uint16
  din_d : UnitDelay  SampleTime=-1
  dout_type : Constant  Value=dout_type
  is_new : simulink/Logic and Bit Operations/Compare To Constant  SystemSampleTime=-1  relop===  const=1  LogicOutDataTypeMode=boolean  ZeroCross=off
  ram : UnitDelay  SampleTime=-1
  ram_data : UnitDelay  SampleTime=-1
  select : Selector  IndexMode=Zero-based  InputPortWidth=2^depth_bits  IndexOptions=Index vector (port)  Indices=[1 3]  OutputSizes=1
  switch : Switch  Criteria=u2 ~= 0
  we_d : UnitDelay  SampleTime=-1
  wr_port : Assignment  IndexMode=Zero-based  IndexOptions=Index vector (port)  Indices=1  OutputSizes=[1 1]
  dout : Outport
  wires:
  DataSpec/1 -> din_d/1, wr_port/2
  we_d/1 -> And/1
  is_new/1 -> And/2
  dout_type/1 -> is_new/1
  ram_data/1 -> Switch1/3
  And/1 -> Switch1/2
  din_d/1 -> Switch1/1
  Switch1/1 -> dout/1
  AddressSpec/1 -> convert/1
  convert/1 -> select/2, wr_port/3
  select/1 -> ram_data/1
  addr/1 -> AddressSpec/1
  we/1 -> we_d/1, switch/2
  din/1 -> DataSpec/1
  ram/1 -> select/1, wr_port/1, switch/3
  switch/1 -> ram/1
  wr_port/1 -> switch/1

== system FaceDet_x4/FaceDetection/DU/SplittedDL3/DelLine4_SPRAM_512x5 ==
  addr : Inport
  din : Inport  Port=2
  we : Inport  Port=3  OutDataTypeStr=boolean
  AddressSpec : SignalSpecification  OutDataTypeStr=fixdt(0,depth_bits,0)  Dimensions=1
  And : Logic  AllPortsSameDT=off  OutDataTypeStr=boolean
  DataSpec : SignalSpecification  OutDataTypeStr=fixdt(0,width_bits,0)  Dimensions=1
  Switch1 : Switch  Criteria=u2 ~= 0
  convert : DataTypeConversion  OutDataTypeStr=uint16
  din_d : UnitDelay  SampleTime=-1
  dout_type : Constant  Value=dout_type
  is_new : simulink/Logic and Bit Operations/Compare To Constant  SystemSampleTime=-1  relop===  const=1  LogicOutDataTypeMode=boolean  ZeroCross=off
  ram : UnitDelay  SampleTime=-1
  ram_data : UnitDelay  SampleTime=-1
  select : Selector  IndexMode=Zero-based  InputPortWidth=2^depth_bits  IndexOptions=Index vector (port)  Indices=[1 3]  OutputSizes=1
  switch : Switch  Criteria=u2 ~= 0
  we_d : UnitDelay  SampleTime=-1
  wr_port : Assignment  IndexMode=Zero-based  IndexOptions=Index vector (port)  Indices=1  OutputSizes=[1 1]
  dout : Outport
  wires:
  wr_port/1 -> switch/1
  switch/1 -> ram/1
  ram/1 -> switch/3, wr_port/1, select/1
  din/1 -> DataSpec/1
  we/1 -> switch/2, we_d/1
  addr/1 -> AddressSpec/1
  select/1 -> ram_data/1
  convert/1 -> wr_port/3, select/2
  AddressSpec/1 -> convert/1
  Switch1/1 -> dout/1
  din_d/1 -> Switch1/1
  And/1 -> Switch1/2
  ram_data/1 -> Switch1/3
  dout_type/1 -> is_new/1
  is_new/1 -> And/2
  we_d/1 -> And/1
  DataSpec/1 -> wr_port/2, din_d/1

== system FaceDet_x4/FaceDetection/DU/SplittedDL3/DelLine5_SPRAM_512x5 ==
  addr : Inport
  din : Inport  Port=2
  we : Inport  Port=3  OutDataTypeStr=boolean
  AddressSpec : SignalSpecification  OutDataTypeStr=fixdt(0,depth_bits,0)  Dimensions=1
  And : Logic  AllPortsSameDT=off  OutDataTypeStr=boolean
  DataSpec : SignalSpecification  OutDataTypeStr=fixdt(0,width_bits,0)  Dimensions=1
  Switch1 : Switch  Criteria=u2 ~= 0
  convert : DataTypeConversion  OutDataTypeStr=uint16
  din_d : UnitDelay  SampleTime=-1
  dout_type : Constant  Value=dout_type
  is_new : simulink/Logic and Bit Operations/Compare To Constant  SystemSampleTime=-1  relop===  const=1  LogicOutDataTypeMode=boolean  ZeroCross=off
  ram : UnitDelay  SampleTime=-1
  ram_data : UnitDelay  SampleTime=-1
  select : Selector  IndexMode=Zero-based  InputPortWidth=2^depth_bits  IndexOptions=Index vector (port)  Indices=[1 3]  OutputSizes=1
  switch : Switch  Criteria=u2 ~= 0
  we_d : UnitDelay  SampleTime=-1
  wr_port : Assignment  IndexMode=Zero-based  IndexOptions=Index vector (port)  Indices=1  OutputSizes=[1 1]
  dout : Outport
  wires:
  DataSpec/1 -> din_d/1, wr_port/2
  we_d/1 -> And/1
  is_new/1 -> And/2
  dout_type/1 -> is_new/1
  ram_data/1 -> Switch1/3
  And/1 -> Switch1/2
  din_d/1 -> Switch1/1
  Switch1/1 -> dout/1
  AddressSpec/1 -> convert/1
  convert/1 -> select/2, wr_port/3
  select/1 -> ram_data/1
  addr/1 -> AddressSpec/1
  we/1 -> we_d/1, switch/2
  din/1 -> DataSpec/1
  ram/1 -> select/1, wr_port/1, switch/3
  switch/1 -> ram/1
  wr_port/1 -> switch/1

== system FaceDet_x4/FaceDetection/DU/SplittedDL3/DelLine6_SPRAM_512x5 ==
  addr : Inport
  din : Inport  Port=2
  we : Inport  Port=3  OutDataTypeStr=boolean
  AddressSpec : SignalSpecification  OutDataTypeStr=fixdt(0,depth_bits,0)  Dimensions=1
  And : Logic  AllPortsSameDT=off  OutDataTypeStr=boolean
  DataSpec : SignalSpecification  OutDataTypeStr=fixdt(0,width_bits,0)  Dimensions=1
  Switch1 : Switch  Criteria=u2 ~= 0
  convert : DataTypeConversion  OutDataTypeStr=uint16
  din_d : UnitDelay  SampleTime=-1
  dout_type : Constant  Value=dout_type
  is_new : simulink/Logic and Bit Operations/Compare To Constant  SystemSampleTime=-1  relop===  const=1  LogicOutDataTypeMode=boolean  ZeroCross=off
  ram : UnitDelay  SampleTime=-1
  ram_data : UnitDelay  SampleTime=-1
  select : Selector  IndexMode=Zero-based  InputPortWidth=2^depth_bits  IndexOptions=Index vector (port)  Indices=[1 3]  OutputSizes=1
  switch : Switch  Criteria=u2 ~= 0
  we_d : UnitDelay  SampleTime=-1
  wr_port : Assignment  IndexMode=Zero-based  IndexOptions=Index vector (port)  Indices=1  OutputSizes=[1 1]
  dout : Outport
  wires:
  DataSpec/1 -> din_d/1, wr_port/2
  we_d/1 -> And/1
  is_new/1 -> And/2
  dout_type/1 -> is_new/1
  ram_data/1 -> Switch1/3
  And/1 -> Switch1/2
  din_d/1 -> Switch1/1
  Switch1/1 -> dout/1
  AddressSpec/1 -> convert/1
  convert/1 -> select/2, wr_port/3
  select/1 -> ram_data/1
  addr/1 -> AddressSpec/1
  we/1 -> we_d/1, switch/2
  din/1 -> DataSpec/1
  ram/1 -> select/1, wr_port/1, switch/3
  switch/1 -> ram/1
  wr_port/1 -> switch/1

== system FaceDet_x4/FaceDetection/DU/SplittedDL3/DelLine7_SPRAM_512x5 ==
  addr : Inport
  din : Inport  Port=2
  we : Inport  Port=3  OutDataTypeStr=boolean
  AddressSpec : SignalSpecification  OutDataTypeStr=fixdt(0,depth_bits,0)  Dimensions=1
  And : Logic  AllPortsSameDT=off  OutDataTypeStr=boolean
  DataSpec : SignalSpecification  OutDataTypeStr=fixdt(0,width_bits,0)  Dimensions=1
  Switch1 : Switch  Criteria=u2 ~= 0
  convert : DataTypeConversion  OutDataTypeStr=uint16
  din_d : UnitDelay  SampleTime=-1
  dout_type : Constant  Value=dout_type
  is_new : simulink/Logic and Bit Operations/Compare To Constant  SystemSampleTime=-1  relop===  const=1  LogicOutDataTypeMode=boolean  ZeroCross=off
  ram : UnitDelay  SampleTime=-1
  ram_data : UnitDelay  SampleTime=-1
  select : Selector  IndexMode=Zero-based  InputPortWidth=2^depth_bits  IndexOptions=Index vector (port)  Indices=[1 3]  OutputSizes=1
  switch : Switch  Criteria=u2 ~= 0
  we_d : UnitDelay  SampleTime=-1
  wr_port : Assignment  IndexMode=Zero-based  IndexOptions=Index vector (port)  Indices=1  OutputSizes=[1 1]
  dout : Outport
  wires:
  wr_port/1 -> switch/1
  switch/1 -> ram/1
  ram/1 -> switch/3, wr_port/1, select/1
  din/1 -> DataSpec/1
  we/1 -> switch/2, we_d/1
  addr/1 -> AddressSpec/1
  select/1 -> ram_data/1
  convert/1 -> wr_port/3, select/2
  AddressSpec/1 -> convert/1
  Switch1/1 -> dout/1
  din_d/1 -> Switch1/1
  And/1 -> Switch1/2
  ram_data/1 -> Switch1/3
  dout_type/1 -> is_new/1
  is_new/1 -> And/2
  we_d/1 -> And/1
  DataSpec/1 -> wr_port/2, din_d/1

== system FaceDet_x4/FaceDetection/FU/AccumulateAllFeatures/UDlyER ==
  note: UnitDelayEnabledResettable
  u : Inport
  E : Inport  Port=2
  R : Inport  Port=3
  FixPt Unit Delay1 : UnitDelay  X0=vinit  SampleTime=tsamp
  ICond : Constant  Value=vinit  OutDataTypeStr=Inherit: Inherit via back propagation
  SwitchEn : MultiPortSwitch  DataPortOrder=Zero-based contiguous  Inputs=2  zeroidx=on
  SwitchRst : MultiPortSwitch  DataPortOrder=Zero-based contiguous  Inputs=2  zeroidx=on
  y : Outport
  wires:
  ICond/1 -> SwitchRst/3  "IVal"
  SwitchRst/1 -> FixPt Unit Delay1/1  "Xnew"
  FixPt Unit Delay1/1 -> SwitchEn/2, y/1  "Xold"
  E/1 -> SwitchEn/1  "Enable"
  u/1 -> SwitchEn/3  "Data"
  SwitchEn/1 -> SwitchRst/2
  R/1 -> SwitchRst/1  "Reset"
